simulink model "Q2"  (R2020b)
settings: Solver=VariableStepAuto  StartTime=0.0  StopTime=10.0  RelTol=1e-3
settings Model: Creator=kushagrakhatwani  LastModifiedBy=kushagrakhatwani

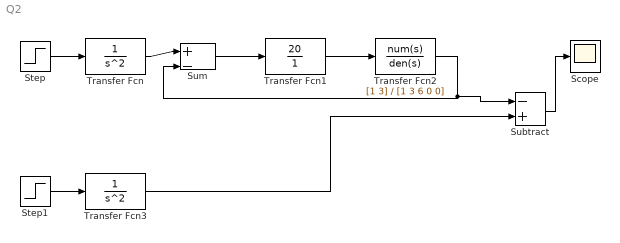
== system Q2 ==
  Scope : Scope
  Step : Step  Time=0  SampleTime=0
  Step1 : Step  Time=0  SampleTime=0
  Subtract : Sum  Inputs=-+
  Sum : Sum  Inputs=|+-
  Transfer Fcn : TransferFcn  Denominator=[1 0 0]
  Transfer Fcn1 : TransferFcn  Numerator=[20]  Denominator=[1]
  Transfer Fcn2 : TransferFcn  Numerator=[1 3]  Denominator=[1 3 6 0 0]
  Transfer Fcn3 : TransferFcn  Denominator=[1 0 0]
  wires:
  Step/1 -> Transfer Fcn/1
  Transfer Fcn/1 -> Sum/1
  Sum/1 -> Transfer Fcn1/1
  Transfer Fcn1/1 -> Transfer Fcn2/1
  Step1/1 -> Transfer Fcn3/1
  Transfer Fcn2/1 -> Sum/2, Subtract/1
  Subtract/1 -> Scope/1
  Transfer Fcn3/1 -> Subtract/2
